simulink model "EHB_speedgoat_R2020a_V1"  (R2020a)
settings: Solver=FixedStepDiscrete  StartTime=0.0  StopTime=inf  FixedStep=0.001  RelTol=1e-3  EnableMultiTasking=on
model workspace (MAT data in the model file):
  A : Simulink.Signal (value not decoded)
  B : Simulink.Signal (value not decoded)
  C : Simulink.Signal (value not decoded)
  D : Simulink.Signal (value not decoded)
  E : Simulink.Signal (value not decoded)
  calin = [-9.96 -7.98 -5.98 -3.99 -1.994 0 1.995 3.992 5.99 7.98 9.97]
  calout = [-10 -8 -6 -4 -2 0 2 4 6 8 10]
symbols that are objects in the model workspace (value not decoded): C, D
undefined symbols (not defined in the file): Com1, none, ts_IO612
libraries: simulink x1436, xpcethercatlib x1223, yisutbxlib_utilities x256, xpcutilitieslib x156, hdlsllib x145, canmsglib x46, speedgoatlib_IO602_4 x11, speedgoatlib_IO611 x7, slrttcplib x4, CanManageLib x3, slrtlib x3, xpcseriallib x2
(part 6 of 30)

== system EHB_speedgoat_R2020a_V1/保留/YS4008/YS4008_M_1 ==
  note: 每路通道4种故障类型，同时最多只能有1个为1（软件保护），当一个通道同时注入超过一种故障时，会自动清除当前通道的所有故障，恢复默认模式。
  note: FIU_SetCH: 0 无故障
      | 1 短路到KL30
      | 2 短路到KL31
      | 4 共轨
      | 8 开路
  note: Rock表示插箱号，一般是0；
      |
      | Slot表示板卡的编号，由板卡上的拨码开关决定；
  FIU_SetCH{1..8} (8 alike) : Constant  Value=0  OutDataTypeStr=Inherit: Inherit via back propagation
  PassWord : Constant  Value=0xAA  OutDataTypeStr=uint8
  Rack : Constant  Value=0  OutDataTypeStr=uint8
  Slot : Constant  OutDataTypeStr=uint8
  YS4008_M : Subsystem
  tag scope: YS4008_M_1=global
  wires:
  PassWord/1 -> YS4008_M/1(PassWord)  "PassWord"
  Rack/1 -> YS4008_M/10(Rack)  "Rack"
  Slot/1 -> YS4008_M/11(Slot)  "Slot"
  FIU_SetCH4/1 -> YS4008_M/5(FIU_SetCH4)  "FIU_SetCH4"
  FIU_SetCH1/1 -> YS4008_M/2(FIU_SetCH1)  "FIU_SetCH1"
  FIU_SetCH8/1 -> YS4008_M/9(FIU_SetCH8)  "FIU_SetCH8"
  FIU_SetCH5/1 -> YS4008_M/6(FIU_SetCH5)  "FIU_SetCH5"
  FIU_SetCH3/1 -> YS4008_M/4(FIU_SetCH3)  "FIU_SetCH3"
  FIU_SetCH2/1 -> YS4008_M/3(FIU_SetCH2)  "FIU_SetCH2"
  FIU_SetCH6/1 -> YS4008_M/7(FIU_SetCH6)  "FIU_SetCH6"
  FIU_SetCH7/1 -> YS4008_M/8(FIU_SetCH7)  "FIU_SetCH7"
  YS4008_M/1(Output) -> [YS4008_M_1]

== system EHB_speedgoat_R2020a_V1/保留/YS4008/YS4008_M_2 ==
  note: Rock表示插箱号，一般是0；
      |
      | Slot表示板卡的编号，由板卡上的拨码开关决定；
  note: FIU_SetCH: 0 无故障
      | 1 短路到KL30
      | 2 短路到KL31
      | 4 共轨
      | 8 开路
  note: 每路通道4种故障类型，同时最多只能有1个为1（软件保护），当一个通道同时注入超过一种故障时，会自动清除当前通道的所有故障，恢复默认模式。
  FIU_SetCH{1..8} (8 alike) : Constant  Value=0  OutDataTypeStr=Inherit: Inherit via back propagation
  PassWord : Constant  Value=0xAA  OutDataTypeStr=uint8
  Rack : Constant  Value=0  OutDataTypeStr=uint8
  Slot : Constant  Value=2  OutDataTypeStr=uint8
  YS4008_M : Subsystem
  tag scope: YS4008_M_2=global
  wires:
  FIU_SetCH6/1 -> YS4008_M/7(FIU_SetCH6)  "FIU_SetCH6"
  FIU_SetCH3/1 -> YS4008_M/4(FIU_SetCH3)  "FIU_SetCH3"
  FIU_SetCH2/1 -> YS4008_M/3(FIU_SetCH2)  "FIU_SetCH2"
  FIU_SetCH1/1 -> YS4008_M/2(FIU_SetCH1)  "FIU_SetCH1"
  FIU_SetCH7/1 -> YS4008_M/8(FIU_SetCH7)  "FIU_SetCH7"
  FIU_SetCH4/1 -> YS4008_M/5(FIU_SetCH4)  "FIU_SetCH4"
  FIU_SetCH5/1 -> YS4008_M/6(FIU_SetCH5)  "FIU_SetCH5"
  FIU_SetCH8/1 -> YS4008_M/9(FIU_SetCH8)  "FIU_SetCH8"
  Slot/1 -> YS4008_M/11(Slot)  "Slot"
  PassWord/1 -> YS4008_M/1(PassWord)  "PassWord"
  Rack/1 -> YS4008_M/10(Rack)  "Rack"
  YS4008_M/1(Output) -> [YS4008_M_2]

== system EHB_speedgoat_R2020a_V1/保留/YS4008/YS4008_M_3 ==
  note: 每路通道4种故障类型，同时最多只能有1个为1（软件保护），当一个通道同时注入超过一种故障时，会自动清除当前通道的所有故障，恢复默认模式。
  note: FIU_SetCH: 0 无故障
      | 1 短路到KL30
      | 2 短路到KL31
      | 4 共轨
      | 8 开路
  note: Rock表示插箱号，一般是0；
      |
      | Slot表示板卡的编号，由板卡上的拨码开关决定；
  FIU_SetCH{1..8} (8 alike) : Constant  Value=0  OutDataTypeStr=Inherit: Inherit via back propagation
  PassWord : Constant  Value=0xAA  OutDataTypeStr=uint8
  Rack : Constant  Value=0  OutDataTypeStr=uint8
  Slot : Constant  Value=3  OutDataTypeStr=uint8
  YS4008_M : Subsystem
  tag scope: YS4008_M_3=global
  wires:
  Rack/1 -> YS4008_M/10(Rack)  "Rack"
  FIU_SetCH8/1 -> YS4008_M/9(FIU_SetCH8)  "FIU_SetCH8"
  Slot/1 -> YS4008_M/11(Slot)  "Slot"
  PassWord/1 -> YS4008_M/1(PassWord)  "PassWord"
  FIU_SetCH5/1 -> YS4008_M/6(FIU_SetCH5)  "FIU_SetCH5"
  FIU_SetCH3/1 -> YS4008_M/4(FIU_SetCH3)  "FIU_SetCH3"
  FIU_SetCH4/1 -> YS4008_M/5(FIU_SetCH4)  "FIU_SetCH4"
  FIU_SetCH2/1 -> YS4008_M/3(FIU_SetCH2)  "FIU_SetCH2"
  FIU_SetCH1/1 -> YS4008_M/2(FIU_SetCH1)  "FIU_SetCH1"
  FIU_SetCH7/1 -> YS4008_M/8(FIU_SetCH7)  "FIU_SetCH7"
  FIU_SetCH6/1 -> YS4008_M/7(FIU_SetCH6)  "FIU_SetCH6"
  YS4008_M/1(Output) -> [YS4008_M_3]

== system EHB_speedgoat_R2020a_V1/保留/YS4008/YS4008_M_4 ==
  note: Rock表示插箱号，一般是0；
      |
      | Slot表示板卡的编号，由板卡上的拨码开关决定；
  note: FIU_SetCH: 0 无故障
      | 1 短路到KL30
      | 2 短路到KL31
      | 4 共轨
      | 8 开路
  note: 每路通道4种故障类型，同时最多只能有1个为1（软件保护），当一个通道同时注入超过一种故障时，会自动清除当前通道的所有故障，恢复默认模式。
  FIU_SetCH{1..8} (8 alike) : Constant  Value=0  OutDataTypeStr=Inherit: Inherit via back propagation
  PassWord : Constant  Value=0xAA  OutDataTypeStr=uint8
  Rack : Constant  Value=0  OutDataTypeStr=uint8
  Slot : Constant  Value=4  OutDataTypeStr=uint8
  YS4008_M1 : Subsystem
  tag scope: YS4008_M_4=global
  wires:
  Rack/1 -> YS4008_M1/10(Rack)  "Rack"
  FIU_SetCH7/1 -> YS4008_M1/8(FIU_SetCH7)  "FIU_SetCH7"
  FIU_SetCH6/1 -> YS4008_M1/7(FIU_SetCH6)  "FIU_SetCH6"
  FIU_SetCH2/1 -> YS4008_M1/3(FIU_SetCH2)  "FIU_SetCH2"
  FIU_SetCH4/1 -> YS4008_M1/5(FIU_SetCH4)  "FIU_SetCH4"
  FIU_SetCH5/1 -> YS4008_M1/6(FIU_SetCH5)  "FIU_SetCH5"
  PassWord/1 -> YS4008_M1/1(PassWord)  "PassWord"
  FIU_SetCH3/1 -> YS4008_M1/4(FIU_SetCH3)  "FIU_SetCH3"
  Slot/1 -> YS4008_M1/11(Slot)  "Slot"
  FIU_SetCH1/1 -> YS4008_M1/2(FIU_SetCH1)  "FIU_SetCH1"
  FIU_SetCH8/1 -> YS4008_M1/9(FIU_SetCH8)  "FIU_SetCH8"
  YS4008_M1/1(Output) -> [YS4008_M_4]

== system EHB_speedgoat_R2020a_V1/保留/YS4008/YS4008_M_5 ==
  note: 每路通道4种故障类型，同时最多只能有1个为1（软件保护），当一个通道同时注入超过一种故障时，会自动清除当前通道的所有故障，恢复默认模式。
  note: FIU_SetCH: 0 无故障
      | 1 短路到KL30
      | 2 短路到KL31
      | 4 共轨
      | 8 开路
  note: Rock表示插箱号，一般是0；
      |
      | Slot表示板卡的编号，由板卡上的拨码开关决定；
  FIU_SetCH{1..8} (8 alike) : Constant  Value=0  OutDataTypeStr=Inherit: Inherit via back propagation
  PassWord : Constant  Value=0xAA  OutDataTypeStr=uint8
  Rack : Constant  Value=0  OutDataTypeStr=uint8
  Slot : Constant  Value=5  OutDataTypeStr=uint8
  YS4008_M : Subsystem
  tag scope: YS4008_M_5=global
  wires:
  FIU_SetCH1/1 -> YS4008_M/2(FIU_SetCH1)  "FIU_SetCH1"
  FIU_SetCH3/1 -> YS4008_M/4(FIU_SetCH3)  "FIU_SetCH3"
  FIU_SetCH5/1 -> YS4008_M/6(FIU_SetCH5)  "FIU_SetCH5"
  Slot/1 -> YS4008_M/11(Slot)  "Slot"
  PassWord/1 -> YS4008_M/1(PassWord)  "PassWord"
  FIU_SetCH4/1 -> YS4008_M/5(FIU_SetCH4)  "FIU_SetCH4"
  FIU_SetCH2/1 -> YS4008_M/3(FIU_SetCH2)  "FIU_SetCH2"
  FIU_SetCH6/1 -> YS4008_M/7(FIU_SetCH6)  "FIU_SetCH6"
  Rack/1 -> YS4008_M/10(Rack)  "Rack"
  FIU_SetCH7/1 -> YS4008_M/8(FIU_SetCH7)  "FIU_SetCH7"
  FIU_SetCH8/1 -> YS4008_M/9(FIU_SetCH8)  "FIU_SetCH8"
  YS4008_M/1(Output) -> [YS4008_M_5]

== system EHB_speedgoat_R2020a_V1/保留/YS4008/YS4008_M_6 ==
  note: Rock表示插箱号，一般是0；
      |
      | Slot表示板卡的编号，由板卡上的拨码开关决定；
  note: FIU_SetCH: 0 无故障
      | 1 短路到KL30
      | 2 短路到KL31
      | 4 共轨
      | 8 开路
  note: 每路通道4种故障类型，同时最多只能有1个为1（软件保护），当一个通道同时注入超过一种故障时，会自动清除当前通道的所有故障，恢复默认模式。
  FIU_SetCH{1..8} (8 alike) : Constant  Value=0  OutDataTypeStr=Inherit: Inherit via back propagation
  PassWord : Constant  Value=0xAA  OutDataTypeStr=uint8
  Rack : Constant  Value=0  OutDataTypeStr=uint8
  Slot : Constant  Value=6  OutDataTypeStr=uint8
  YS4008_M : Subsystem
  tag scope: YS4008_M_6=global
  wires:
  FIU_SetCH7/1 -> YS4008_M/8(FIU_SetCH7)  "FIU_SetCH7"
  Slot/1 -> YS4008_M/11(Slot)  "Slot"
  FIU_SetCH6/1 -> YS4008_M/7(FIU_SetCH6)  "FIU_SetCH6"
  FIU_SetCH2/1 -> YS4008_M/3(FIU_SetCH2)  "FIU_SetCH2"
  FIU_SetCH4/1 -> YS4008_M/5(FIU_SetCH4)  "FIU_SetCH4"
  Rack/1 -> YS4008_M/10(Rack)  "Rack"
  FIU_SetCH3/1 -> YS4008_M/4(FIU_SetCH3)  "FIU_SetCH3"
  FIU_SetCH5/1 -> YS4008_M/6(FIU_SetCH5)  "FIU_SetCH5"
  FIU_SetCH8/1 -> YS4008_M/9(FIU_SetCH8)  "FIU_SetCH8"
  FIU_SetCH1/1 -> YS4008_M/2(FIU_SetCH1)  "FIU_SetCH1"
  PassWord/1 -> YS4008_M/1(PassWord)  "PassWord"
  YS4008_M/1(Output) -> [YS4008_M_6]

== system EHB_speedgoat_R2020a_V1/保留/YS7501_M/HVRealy_Set ==
  RLY1 : Inport
  RLY2 : Inport  Port=2
  RLY3 : Inport  Port=3
  RLY4 : Inport  Port=4
  RLY5 : Inport  Port=5
  RLY6 : Inport  Port=6
  RLY7 : Inport  Port=7
  RLY8 : Inport  Port=8
  RLY9 : Inport  Port=9
  RLY10 : Inport  Port=10
  RLY11 : Inport  Port=11
  RLY12 : Inport  Port=12
  RLY13 : Inport  Port=13
  RLY14 : Inport  Port=14
  RLY15 : Inport  Port=15
  RLY16 : Inport  Port=16
  Trigger : TriggerPort  VariantControl=(inherit)  PortDimensions=1
  CAN Pack1 : canmsglib/CAN Pack  MsgList=(none)  MsgName=YS7501_M  MsgIDType=Standard (11-bit identifier)  MsgIdentifier=1856  MsgLength=8  Remote=off  ApplyMinMax=off  BusOutput=on  SignalInfo={ 'Rly1', '8', '1', 'BE', 'unsigned', 'Standard', '0', '1', '0', '0', '1'; 'Rly10', '17', '1', 'BE', 'unsigned', 'Standard', '0', '1', '0', '0', '1'; 'Rly11', '18', '1', 'BE', 'unsigned', 'Standard', '0', '1', '0', '0', '1'; 'Rly12', '19', '1', 'BE', 'unsigned', 'Standard', '0', '1', '0', '0', '1'; 'Rly13', '20', '1', 'BE', 'unsigned', 'Standard', '0', '1', '0', '0', '1'; 'Rly14', '21', '1', 'BE', 'unsigned', 'Standard', '0', '1', '0', '0', '1'; 'Rly15', '22', '1', 'BE', 'unsigned', 'Standard', '0', '1', '0', '0', '1'; 'Rly16', '23', '1', 'BE', 'unsigned', 'Standard', '0', '1', '0', '0', '1'; 'Rly2', '9', '1', 'BE', 'unsigned', 'Standard', '0', '1', '0', '0', '1'; 'Rly3', '10', '1', 'BE', 'unsigned', 'Standard', '0', '1', '0', '0', '1'; 'Rly4', '11', '1', 'BE', 'unsigned', 'Standard', '0', '1', '0', '0', '1'; 'Rly5', '12', '1', 'BE', 'unsigned', 'Standard', '0', '1', '0', '0', '1'; 'Rly6', '13', '1', 'BE', 'unsigned', 'Standard', '0', '1', '0', '0', '1'; 'Rly7', '14', '1', 'BE', 'unsigned', 'Standard', '0', '1', '0', '0', '1'; 'Rly8', '15', '1', 'BE', 'unsigned', 'Standard', '0', '1', '0', '0', '1'; 'Rly9', '16', '1', 'BE', 'unsigned', 'Standard', '0', '1', '0', '0', '1'; 'Rly_en', '0', '1', 'BE', 'unsigned', 'Standard', '0', '1', '0', '0', '1' }
      settings: SourceProductBaseCode=ME,VN  DataFormat=manually specified signals
  CANDataPack_ToUDP : Subsystem
  Constant : Constant
  Output : Outport
  wires:
  CAN Pack1/1 -> CANDataPack_ToUDP/1(In1)
  RLY1/1 -> CAN Pack1/1
  RLY2/1 -> CAN Pack1/9
  RLY3/1 -> CAN Pack1/10
  RLY4/1 -> CAN Pack1/11
  RLY5/1 -> CAN Pack1/12
  RLY6/1 -> CAN Pack1/13
  RLY7/1 -> CAN Pack1/14
  RLY8/1 -> CAN Pack1/15
  RLY9/1 -> CAN Pack1/16
  RLY14/1 -> CAN Pack1/6
  RLY13/1 -> CAN Pack1/5
  RLY12/1 -> CAN Pack1/4
  RLY11/1 -> CAN Pack1/3
  RLY10/1 -> CAN Pack1/2
  RLY15/1 -> CAN Pack1/7
  RLY16/1 -> CAN Pack1/8
  Constant/1 -> CAN Pack1/17
  CANDataPack_ToUDP/1(Output) -> Output/1

== system EHB_speedgoat_R2020a_V1/CAN_Send/CAN Transmit/VCU_Msg/VCU_BrakingRequest_0x120 ==
  VCU_BrakingRequest : Inport
  Enable : EnablePort
  Trigger : TriggerPort  VariantControl=Variant
  Bus Selector : BusSelector  OutputSignals=Brake_AimPressure,BrakingEnable,ParkingBrakeActive
  CAN Pack : canmsglib/CAN Pack  CANdbFile=F:\湖大艾盛\wushuadianji_20230612.dbc  MsgList=VCU_BrakingRequest  MsgName=VCU_BrakingRequest  MsgIDType=Standard (11-bit identifier)  MsgIdentifier=288  MsgLength=8  Remote=off  ApplyMinMax=off  BusOutput=on  SignalInfo={'Brake_AimPressure','8','8','BE','unsigned','Standard','0','0.1','0','-Inf','Inf';'BrakingEnable','0','4','BE','unsigned','Standard','0','1','0','-Inf','Inf';'ParkingBrakeActive','4','4','BE','unsigned','Standard','0','1','0','-Inf','Inf'}
      settings: SourceProductBaseCode=ME,VN  DataFormat=CANdb specified signals
  CAN Write : speedgoatlib_IO602_4/Legacy/CAN Write  id=1  ts=-1  channel=1  messageType=CAN  BusInput=on  enableStatusPort=off  canType=CAN (HS)  initValues=[602 1 -1 0 1 1 0 1]
      settings: SourceProductName=Simulink Real-Time: Speedgoat I/O Blockset
  sigSource1 : Subsystem
  sigSource2 : Subsystem
  sigSource3 : Subsystem
  wires:
  VCU_BrakingRequest/1 -> Bus Selector/1
  Bus Selector/1 -> sigSource1/1(InputSignal)  "<Brake_AimPressure>"
  sigSource1/1(OutputSignal) -> CAN Pack/1
  Bus Selector/2 -> sigSource2/1(InputSignal)  "<BrakingEnable>"
  sigSource2/1(OutputSignal) -> CAN Pack/2
  Bus Selector/3 -> sigSource3/1(InputSignal)  "<ParkingBrakeActive>"
  sigSource3/1(OutputSignal) -> CAN Pack/3
  CAN Pack/1 -> CAN Write/1

== system EHB_speedgoat_R2020a_V1/CAN_Send/Signal/CAN_Msg_VCU/VCU_BrakingRequest_0x120 ==
  Brake_AimPressure : Constant  Value=0
  BrakingEnable : Constant  Value=0
  Bus Creator : BusCreator  Inputs=3
  ParkingBrakeActive : Constant  Value=0
  dtc1 : DataTypeConversion
  dtc2 : DataTypeConversion
  dtc3 : DataTypeConversion
  VCU_BrakingRequest_0x120 : Outport
  wires:
  dtc1/1 -> Bus Creator/1  "Brake_AimPressure"
  Brake_AimPressure/1 -> dtc1/1  "Brake_AimPressure"
  dtc2/1 -> Bus Creator/2  "BrakingEnable"
  BrakingEnable/1 -> dtc2/1  "BrakingEnable"
  dtc3/1 -> Bus Creator/3  "ParkingBrakeActive"
  ParkingBrakeActive/1 -> dtc3/1  "ParkingBrakeActive"
  Bus Creator/1 -> VCU_BrakingRequest_0x120/1  "VCU_BrakingRequest_0x120"

== system EHB_speedgoat_R2020a_V1/CAN_Send/Trigger/Trigger_VCU_Msg/Trigger_VCU_BrakingRequest_0x120 ==
  note: 发送触发方式的拓展：
      | 1、循环周期发送(包括丢帧方式)；
      | 2、手动触发发送(增加调试模块)；
      | 3、待拓展模式；
  ConditionalTrigger : Ground
  Cycle : Subsystem
  Kick : Subsystem
  KickValueChange : Subsystem
      settings: OpenFcn=|
      | KickValuePath =[gcs,'/Kick/KickValue'];
      | KickValueTmp = str2num(get_param(KickValuePath,'Value'));
      | if KickValueTmp == 1
      | set_param(KickValuePath,'Value','0');
      | else
      | set_param(KickValuePath,'Value','1');
      | end
      | masKicks = Simulink.Mask.get(gcb);
      | DispKicks = sprintf('disp("KicksValue:%s")',get_param(KickValuePath,'Value'));
      | masKicks.Display = DispKicks;
      mask Display: disp("KicksValue:1")
  ModeSelect : Constant  Value=ModeSelect  SampleTime=-1
  Multiport Switch : MultiPortSwitch
  Out1 : Outport  VectorParamsAs1DForOutWhenUnconnected=off
  wires:
  ConditionalTrigger/1 -> Multiport Switch/4
  Multiport Switch/1 -> Out1/1
  ModeSelect/1 -> Multiport Switch/1
  Cycle/1(Out1) -> Multiport Switch/2
  Kick/1(Out1) -> Multiport Switch/3

== system EHB_speedgoat_R2020a_V1/PowerCtrl/PowerCtrl/CANOpenInit1/CANDataPack_ToUDP ==
  In1 : Inport
  "Bit Packing " : xpcutilitieslib/Bit Packing   MaskBitPatterns={[7],[6],[4 5],[0:3]}  MaskPackDataType=uint8  MaskPackDataSize=[1]
      settings: SourceProductBaseCode=XP
  Bit Slice : hdlsllib/Logic and Bit Operations/Bit Slice  lidx=3  ridx=0
      settings: SourceProductBaseCode=SL
  Bus Selector : BusSelector  OutputSignals=Extended,Length,Remote,ID,Data
  "Byte Packing " : xpcutilitieslib/Byte Packing   MaskPackedDataType=uint8  MaskUnpackedDataTypes={'uint32'}  MaskAlignment=1
  "Byte Reversal " : xpcutilitieslib/Byte Reversal   numInp=1
      settings: SourceProductBaseCode=XP
  Constant1 : Constant  Value=[0 0]
  Data Type Conversion1 : DataTypeConversion  OutDataTypeStr=boolean
  Data Type Conversion2 : DataTypeConversion  OutDataTypeStr=uint8
  Data Type Conversion9 : DataTypeConversion  OutDataTypeStr=boolean
  Mux : Mux  Inputs=3
  Output : Outport
  wires:
  Bus Selector/5 -> Mux/3  "<Data>"
  "Bit Packing "/1 -> Mux/1  "YS5002_PowerSet"
  Bus Selector/2 -> Data Type Conversion2/1  "<Length>"
  Bus Selector/4 -> "Byte Reversal "/1  "<ID>"
  In1/1 -> Bus Selector/1
  Bus Selector/1 -> Data Type Conversion9/1  "<Extended>"
  Bus Selector/3 -> Data Type Conversion1/1  "<Remote>"
  Data Type Conversion9/1 -> "Bit Packing "/1
  "Byte Reversal "/1 -> "Byte Packing "/1
  Bit Slice/1 -> "Bit Packing "/4
  "Byte Packing "/1 -> Mux/2
  Constant1/1 -> "Bit Packing "/3
  Mux/1 -> Output/1
  Data Type Conversion2/1 -> Bit Slice/1
  Data Type Conversion1/1 -> "Bit Packing "/2

== system EHB_speedgoat_R2020a_V1/PowerCtrl/PowerCtrl/CurrSet1/CANDataPack_ToUDP ==
  In1 : Inport
  "Bit Packing " : xpcutilitieslib/Bit Packing   MaskBitPatterns={[7],[6],[4 5],[0:3]}  MaskPackDataType=uint8  MaskPackDataSize=[1]
      settings: SourceProductBaseCode=XP
  Bit Slice : hdlsllib/Logic and Bit Operations/Bit Slice  lidx=3  ridx=0
      settings: SourceProductBaseCode=SL
  Bus Selector : BusSelector  OutputSignals=Extended,Length,Remote,ID,Data
  "Byte Packing " : xpcutilitieslib/Byte Packing   MaskPackedDataType=uint8  MaskUnpackedDataTypes={'uint32'}  MaskAlignment=1
  "Byte Reversal " : xpcutilitieslib/Byte Reversal   numInp=1
      settings: SourceProductBaseCode=XP
  Constant1 : Constant  Value=[0 0]
  Data Type Conversion1 : DataTypeConversion  OutDataTypeStr=boolean
  Data Type Conversion2 : DataTypeConversion  OutDataTypeStr=uint8
  Data Type Conversion9 : DataTypeConversion  OutDataTypeStr=boolean
  Mux : Mux  Inputs=3
  Output : Outport
  wires:
  Bus Selector/5 -> Mux/3  "<Data>"
  "Bit Packing "/1 -> Mux/1  "YS5002_PowerSet"
  Bus Selector/2 -> Data Type Conversion2/1  "<Length>"
  Bus Selector/4 -> "Byte Reversal "/1  "<ID>"
  In1/1 -> Bus Selector/1
  Bus Selector/1 -> Data Type Conversion9/1  "<Extended>"
  Bus Selector/3 -> Data Type Conversion1/1  "<Remote>"
  Data Type Conversion9/1 -> "Bit Packing "/1
  "Byte Reversal "/1 -> "Byte Packing "/1
  Bit Slice/1 -> "Bit Packing "/4
  "Byte Packing "/1 -> Mux/2
  Constant1/1 -> "Bit Packing "/3
  Mux/1 -> Output/1
  Data Type Conversion2/1 -> Bit Slice/1
  Data Type Conversion1/1 -> "Bit Packing "/2

== system EHB_speedgoat_R2020a_V1/PowerCtrl/PowerCtrl/Enable1/CANDataPack_ToUDP ==
  In1 : Inport
  "Bit Packing " : xpcutilitieslib/Bit Packing   MaskBitPatterns={[7],[6],[4 5],[0:3]}  MaskPackDataType=uint8  MaskPackDataSize=[1]
      settings: SourceProductBaseCode=XP
  Bit Slice : hdlsllib/Logic and Bit Operations/Bit Slice  lidx=3  ridx=0
      settings: SourceProductBaseCode=SL
  Bus Selector : BusSelector  OutputSignals=Extended,Length,Remote,ID,Data
  "Byte Packing " : xpcutilitieslib/Byte Packing   MaskPackedDataType=uint8  MaskUnpackedDataTypes={'uint32'}  MaskAlignment=1
  "Byte Reversal " : xpcutilitieslib/Byte Reversal   numInp=1
      settings: SourceProductBaseCode=XP
  Constant1 : Constant  Value=[0 0]
  Data Type Conversion1 : DataTypeConversion  OutDataTypeStr=boolean
  Data Type Conversion2 : DataTypeConversion  OutDataTypeStr=uint8
  Data Type Conversion9 : DataTypeConversion  OutDataTypeStr=boolean
  Mux : Mux  Inputs=3
  Output : Outport
  wires:
  Bus Selector/5 -> Mux/3  "<Data>"
  "Bit Packing "/1 -> Mux/1  "YS5002_PowerSet"
  Bus Selector/2 -> Data Type Conversion2/1  "<Length>"
  Bus Selector/4 -> "Byte Reversal "/1  "<ID>"
  In1/1 -> Bus Selector/1
  Bus Selector/1 -> Data Type Conversion9/1  "<Extended>"
  Bus Selector/3 -> Data Type Conversion1/1  "<Remote>"
  Data Type Conversion9/1 -> "Bit Packing "/1
  "Byte Reversal "/1 -> "Byte Packing "/1
  Bit Slice/1 -> "Bit Packing "/4
  "Byte Packing "/1 -> Mux/2
  Constant1/1 -> "Bit Packing "/3
  Mux/1 -> Output/1
  Data Type Conversion2/1 -> Bit Slice/1
  Data Type Conversion1/1 -> "Bit Packing "/2

== system EHB_speedgoat_R2020a_V1/PowerCtrl/PowerCtrl/PowerPosSet1/CANDataPack_ToUDP ==
  In1 : Inport
  "Bit Packing " : xpcutilitieslib/Bit Packing   MaskBitPatterns={[7],[6],[4 5],[0:3]}  MaskPackDataType=uint8  MaskPackDataSize=[1]
      settings: SourceProductBaseCode=XP
  Bit Slice : hdlsllib/Logic and Bit Operations/Bit Slice  lidx=3  ridx=0
      settings: SourceProductBaseCode=SL
  Bus Selector : BusSelector  OutputSignals=Extended,Length,Remote,ID,Data
  "Byte Packing " : xpcutilitieslib/Byte Packing   MaskPackedDataType=uint8  MaskUnpackedDataTypes={'uint32'}  MaskAlignment=1
  "Byte Reversal " : xpcutilitieslib/Byte Reversal   numInp=1
      settings: SourceProductBaseCode=XP
  Constant1 : Constant  Value=[0 0]
  Data Type Conversion1 : DataTypeConversion  OutDataTypeStr=boolean
  Data Type Conversion2 : DataTypeConversion  OutDataTypeStr=uint8
  Data Type Conversion9 : DataTypeConversion  OutDataTypeStr=boolean
  Mux : Mux  Inputs=3
  Output : Outport
  wires:
  Bus Selector/5 -> Mux/3  "<Data>"
  "Bit Packing "/1 -> Mux/1  "YS5002_PowerSet"
  Bus Selector/2 -> Data Type Conversion2/1  "<Length>"
  Bus Selector/4 -> "Byte Reversal "/1  "<ID>"
  In1/1 -> Bus Selector/1
  Bus Selector/1 -> Data Type Conversion9/1  "<Extended>"
  Bus Selector/3 -> Data Type Conversion1/1  "<Remote>"
  Data Type Conversion9/1 -> "Bit Packing "/1
  "Byte Reversal "/1 -> "Byte Packing "/1
  Bit Slice/1 -> "Bit Packing "/4
  "Byte Packing "/1 -> Mux/2
  Constant1/1 -> "Bit Packing "/3
  Mux/1 -> Output/1
  Data Type Conversion2/1 -> Bit Slice/1
  Data Type Conversion1/1 -> "Bit Packing "/2

== system EHB_speedgoat_R2020a_V1/PowerCtrl/PowerCtrl/VoltSet1/CANDataPack_ToUDP ==
  In1 : Inport
  "Bit Packing " : xpcutilitieslib/Bit Packing   MaskBitPatterns={[7],[6],[4 5],[0:3]}  MaskPackDataType=uint8  MaskPackDataSize=[1]
      settings: SourceProductBaseCode=XP
  Bit Slice : hdlsllib/Logic and Bit Operations/Bit Slice  lidx=3  ridx=0
      settings: SourceProductBaseCode=SL
  Bus Selector : BusSelector  OutputSignals=Extended,Length,Remote,ID,Data
  "Byte Packing " : xpcutilitieslib/Byte Packing   MaskPackedDataType=uint8  MaskUnpackedDataTypes={'uint32'}  MaskAlignment=1
  "Byte Reversal " : xpcutilitieslib/Byte Reversal   numInp=1
      settings: SourceProductBaseCode=XP
  Constant1 : Constant  Value=[0 0]
  Data Type Conversion1 : DataTypeConversion  OutDataTypeStr=boolean
  Data Type Conversion2 : DataTypeConversion  OutDataTypeStr=uint8
  Data Type Conversion9 : DataTypeConversion  OutDataTypeStr=boolean
  Mux : Mux  Inputs=3
  Output : Outport
  wires:
  Bus Selector/5 -> Mux/3  "<Data>"
  "Bit Packing "/1 -> Mux/1  "YS5002_PowerSet"
  Bus Selector/2 -> Data Type Conversion2/1  "<Length>"
  Bus Selector/4 -> "Byte Reversal "/1  "<ID>"
  In1/1 -> Bus Selector/1
  Bus Selector/1 -> Data Type Conversion9/1  "<Extended>"
  Bus Selector/3 -> Data Type Conversion1/1  "<Remote>"
  Data Type Conversion9/1 -> "Bit Packing "/1
  "Byte Reversal "/1 -> "Byte Packing "/1
  Bit Slice/1 -> "Bit Packing "/4
  "Byte Packing "/1 -> Mux/2
  Constant1/1 -> "Bit Packing "/3
  Mux/1 -> Output/1
  Data Type Conversion2/1 -> Bit Slice/1
  Data Type Conversion1/1 -> "Bit Packing "/2

== system EHB_speedgoat_R2020a_V1/TIF_04/CB2020_1/DAC1/dp2c CH1 ==
  dac_value : Inport
  dac_value_calibrate : Inport  Port=2
  Add : Sum
  Add1 : Sum
  Constant : Constant  Value=0
  Data Type Conversion : DataTypeConversion  OutDataTypeStr=int16
  Gain : Gain  Gain=32767/15
  Gain1 : Gain
  Saturation : Saturate  UpperLimit=12  LowerLimit=-12
  cmd_value : Outport
  wires:
  Gain/1 -> Add1/1
  Saturation/1 -> Add/1
  dac_value_calibrate/1 -> Add1/2
  dac_value/1 -> Gain1/1
  Constant/1 -> Add/2
  Add/1 -> Gain/1
  Data Type Conversion/1 -> cmd_value/1
  Add1/1 -> Data Type Conversion/1
  Gain1/1 -> Saturation/1

== system EHB_speedgoat_R2020a_V1/TIF_04/CB2020_2/DAC/dp2c CH1 ==
  dac_value : Inport
  dac_value_calibrate : Inport  Port=2
  Add : Sum
  Add1 : Sum
  Constant : Constant  Value=0
  Data Type Conversion : DataTypeConversion
  Gain : Gain  Gain=32767/15
  Gain1 : Gain
  Saturation : Saturate  UpperLimit=12  LowerLimit=-12
  cmd_value : Outport
  wires:
  Gain/1 -> Add1/1
  Saturation/1 -> Add/1
  dac_value_calibrate/1 -> Add1/2
  dac_value/1 -> Gain1/1
  Constant/1 -> Add/2
  Add/1 -> Gain/1
  Data Type Conversion/1 -> cmd_value/1
  Add1/1 -> Data Type Conversion/1
  Gain1/1 -> Saturation/1

== system EHB_speedgoat_R2020a_V1/TIF_04/CB2020_2/DAC/dp2c CH10 ==
  dac_value : Inport
  dac_value_calibrate : Inport  Port=2
  Add : Sum
  Add1 : Sum
  Constant : Constant  Value=0
  Data Type Conversion : DataTypeConversion
  Gain : Gain  Gain=32767/15
  Gain1 : Gain
  Saturation : Saturate  UpperLimit=12  LowerLimit=-12
  cmd_value : Outport
  wires:
  Gain/1 -> Add1/1
  Saturation/1 -> Add/1
  dac_value_calibrate/1 -> Add1/2
  dac_value/1 -> Gain1/1
  Constant/1 -> Add/2
  Add/1 -> Gain/1
  Data Type Conversion/1 -> cmd_value/1
  Add1/1 -> Data Type Conversion/1
  Gain1/1 -> Saturation/1

== system EHB_speedgoat_R2020a_V1/TIF_04/CB2020_2/DAC/dp2c CH11 ==
  dac_value : Inport
  dac_value_calibrate : Inport  Port=2
  Add : Sum
  Add1 : Sum
  Constant : Constant  Value=0
  Data Type Conversion : DataTypeConversion
  Gain : Gain  Gain=32767/15
  Gain1 : Gain
  Saturation : Saturate  UpperLimit=12  LowerLimit=-12
  cmd_value : Outport
  wires:
  Gain/1 -> Add1/1
  Saturation/1 -> Add/1
  dac_value_calibrate/1 -> Add1/2
  dac_value/1 -> Gain1/1
  Constant/1 -> Add/2
  Add/1 -> Gain/1
  Data Type Conversion/1 -> cmd_value/1
  Add1/1 -> Data Type Conversion/1
  Gain1/1 -> Saturation/1

== system EHB_speedgoat_R2020a_V1/TIF_04/CB2020_2/DAC/dp2c CH12 ==
  dac_value : Inport
  dac_value_calibrate : Inport  Port=2
  Add : Sum
  Add1 : Sum
  Constant : Constant  Value=0
  Data Type Conversion : DataTypeConversion
  Gain : Gain  Gain=32767/15
  Gain1 : Gain
  Saturation : Saturate  UpperLimit=12  LowerLimit=-12
  cmd_value : Outport
  wires:
  Gain/1 -> Add1/1
  Saturation/1 -> Add/1
  dac_value_calibrate/1 -> Add1/2
  dac_value/1 -> Gain1/1
  Constant/1 -> Add/2
  Add/1 -> Gain/1
  Data Type Conversion/1 -> cmd_value/1
  Add1/1 -> Data Type Conversion/1
  Gain1/1 -> Saturation/1

== system EHB_speedgoat_R2020a_V1/TIF_04/CB2020_2/DAC/dp2c CH13 ==
  dac_value : Inport
  dac_value_calibrate : Inport  Port=2
  Add : Sum
  Add1 : Sum
  Constant : Constant  Value=0
  Data Type Conversion : DataTypeConversion
  Gain : Gain  Gain=32767/15
  Gain1 : Gain
  Saturation : Saturate  UpperLimit=12  LowerLimit=-12
  cmd_value : Outport
  wires:
  Gain/1 -> Add1/1
  Saturation/1 -> Add/1
  dac_value_calibrate/1 -> Add1/2
  dac_value/1 -> Gain1/1
  Constant/1 -> Add/2
  Add/1 -> Gain/1
  Data Type Conversion/1 -> cmd_value/1
  Add1/1 -> Data Type Conversion/1
  Gain1/1 -> Saturation/1

== system EHB_speedgoat_R2020a_V1/TIF_04/CB2020_2/DAC/dp2c CH14 ==
  dac_value : Inport
  dac_value_calibrate : Inport  Port=2
  Add : Sum
  Add1 : Sum
  Constant : Constant  Value=0
  Data Type Conversion : DataTypeConversion
  Gain : Gain  Gain=32767/15
  Gain1 : Gain
  Saturation : Saturate  UpperLimit=12  LowerLimit=-12
  cmd_value : Outport
  wires:
  Gain/1 -> Add1/1
  Saturation/1 -> Add/1
  dac_value_calibrate/1 -> Add1/2
  dac_value/1 -> Gain1/1
  Constant/1 -> Add/2
  Add/1 -> Gain/1
  Data Type Conversion/1 -> cmd_value/1
  Add1/1 -> Data Type Conversion/1
  Gain1/1 -> Saturation/1

== system EHB_speedgoat_R2020a_V1/TIF_04/CB2020_2/DAC/dp2c CH15 ==
  dac_value : Inport
  dac_value_calibrate : Inport  Port=2
  Add : Sum
  Add1 : Sum
  Constant : Constant  Value=0
  Data Type Conversion : DataTypeConversion
  Gain : Gain  Gain=32767/15
  Gain1 : Gain
  Saturation : Saturate  UpperLimit=12  LowerLimit=-12
  cmd_value : Outport
  wires:
  Gain/1 -> Add1/1
  Saturation/1 -> Add/1
  dac_value_calibrate/1 -> Add1/2
  dac_value/1 -> Gain1/1
  Constant/1 -> Add/2
  Add/1 -> Gain/1
  Data Type Conversion/1 -> cmd_value/1
  Add1/1 -> Data Type Conversion/1
  Gain1/1 -> Saturation/1

== system EHB_speedgoat_R2020a_V1/TIF_04/CB2020_2/DAC/dp2c CH16 ==
  dac_value : Inport
  dac_value_calibrate : Inport  Port=2
  Add : Sum
  Add1 : Sum
  Constant : Constant  Value=0
  Data Type Conversion : DataTypeConversion
  Gain : Gain  Gain=32767/15
  Gain1 : Gain
  Saturation : Saturate  UpperLimit=12  LowerLimit=-12
  cmd_value : Outport
  wires:
  Gain/1 -> Add1/1
  Saturation/1 -> Add/1
  dac_value_calibrate/1 -> Add1/2
  dac_value/1 -> Gain1/1
  Constant/1 -> Add/2
  Add/1 -> Gain/1
  Data Type Conversion/1 -> cmd_value/1
  Add1/1 -> Data Type Conversion/1
  Gain1/1 -> Saturation/1

== system EHB_speedgoat_R2020a_V1/TIF_04/CB2020_2/DAC/dp2c CH17 ==
  dac_value : Inport
  dac_value_calibrate : Inport  Port=2
  Add : Sum
  Add1 : Sum
  Constant : Constant  Value=0
  Data Type Conversion : DataTypeConversion
  Gain : Gain  Gain=32767/10
  Gain1 : Gain
  Saturation : Saturate  UpperLimit=10  LowerLimit=-10
  cmd_value : Outport
  wires:
  Gain/1 -> Add1/1
  Saturation/1 -> Add/1
  dac_value_calibrate/1 -> Add1/2
  dac_value/1 -> Gain1/1
  Constant/1 -> Add/2
  Add/1 -> Gain/1
  Data Type Conversion/1 -> cmd_value/1
  Add1/1 -> Data Type Conversion/1
  Gain1/1 -> Saturation/1

== system EHB_speedgoat_R2020a_V1/TIF_04/CB2020_2/DAC/dp2c CH18 ==
  dac_value : Inport
  dac_value_calibrate : Inport  Port=2
  Add : Sum
  Add1 : Sum
  Constant : Constant  Value=0
  Data Type Conversion : DataTypeConversion
  Gain : Gain  Gain=32767/10
  Gain1 : Gain
  Saturation : Saturate  UpperLimit=10  LowerLimit=-10
  cmd_value : Outport
  wires:
  Gain/1 -> Add1/1
  Saturation/1 -> Add/1
  dac_value_calibrate/1 -> Add1/2
  dac_value/1 -> Gain1/1
  Constant/1 -> Add/2
  Add/1 -> Gain/1
  Data Type Conversion/1 -> cmd_value/1
  Add1/1 -> Data Type Conversion/1
  Gain1/1 -> Saturation/1

== system EHB_speedgoat_R2020a_V1/TIF_04/CB2020_2/DAC/dp2c CH19 ==
  dac_value : Inport
  dac_value_calibrate : Inport  Port=2
  Add : Sum
  Add1 : Sum
  Constant : Constant  Value=0
  Data Type Conversion : DataTypeConversion
  Gain : Gain  Gain=32767/10
  Gain1 : Gain
  Saturation : Saturate  UpperLimit=10  LowerLimit=-10
  cmd_value : Outport
  wires:
  Gain/1 -> Add1/1
  Saturation/1 -> Add/1
  dac_value_calibrate/1 -> Add1/2
  dac_value/1 -> Gain1/1
  Constant/1 -> Add/2
  Add/1 -> Gain/1
  Data Type Conversion/1 -> cmd_value/1
  Add1/1 -> Data Type Conversion/1
  Gain1/1 -> Saturation/1

== system EHB_speedgoat_R2020a_V1/TIF_04/CB2020_2/DAC/dp2c CH2 ==
  dac_value : Inport
  dac_value_calibrate : Inport  Port=2
  Add : Sum
  Add1 : Sum
  Constant : Constant  Value=0
  Data Type Conversion : DataTypeConversion
  Gain : Gain  Gain=32767/15
  Gain1 : Gain
  Saturation : Saturate  UpperLimit=12  LowerLimit=-12
  cmd_value : Outport
  wires:
  Gain/1 -> Add1/1
  Saturation/1 -> Add/1
  dac_value_calibrate/1 -> Add1/2
  dac_value/1 -> Gain1/1
  Constant/1 -> Add/2
  Add/1 -> Gain/1
  Data Type Conversion/1 -> cmd_value/1
  Add1/1 -> Data Type Conversion/1
  Gain1/1 -> Saturation/1

== system EHB_speedgoat_R2020a_V1/TIF_04/CB2020_2/DAC/dp2c CH20 ==
  dac_value : Inport
  dac_value_calibrate : Inport  Port=2
  Add : Sum
  Add1 : Sum
  Constant : Constant  Value=0
  Data Type Conversion : DataTypeConversion
  Gain : Gain  Gain=32767/10
  Gain1 : Gain
  Saturation : Saturate  UpperLimit=10  LowerLimit=-10
  cmd_value : Outport
  wires:
  Gain/1 -> Add1/1
  Saturation/1 -> Add/1
  dac_value_calibrate/1 -> Add1/2
  dac_value/1 -> Gain1/1
  Constant/1 -> Add/2
  Add/1 -> Gain/1
  Data Type Conversion/1 -> cmd_value/1
  Add1/1 -> Data Type Conversion/1
  Gain1/1 -> Saturation/1

== system EHB_speedgoat_R2020a_V1/TIF_04/CB2020_2/DAC/dp2c CH3 ==
  dac_value : Inport
  dac_value_calibrate : Inport  Port=2
  Add : Sum
  Add1 : Sum
  Constant : Constant  Value=0
  Data Type Conversion : DataTypeConversion
  Gain : Gain  Gain=32767/15
  Gain1 : Gain
  Saturation : Saturate  UpperLimit=12  LowerLimit=-12
  cmd_value : Outport
  wires:
  Gain/1 -> Add1/1
  Saturation/1 -> Add/1
  dac_value_calibrate/1 -> Add1/2
  dac_value/1 -> Gain1/1
  Constant/1 -> Add/2
  Add/1 -> Gain/1
  Data Type Conversion/1 -> cmd_value/1
  Add1/1 -> Data Type Conversion/1
  Gain1/1 -> Saturation/1

== system EHB_speedgoat_R2020a_V1/TIF_04/CB2020_2/DAC/dp2c CH4 ==
  dac_value : Inport
  dac_value_calibrate : Inport  Port=2
  Add : Sum
  Add1 : Sum
  Constant : Constant  Value=0
  Data Type Conversion : DataTypeConversion
  Gain : Gain  Gain=32767/15
  Gain1 : Gain
  Saturation : Saturate  UpperLimit=12  LowerLimit=-12
  cmd_value : Outport
  wires:
  Gain/1 -> Add1/1
  Saturation/1 -> Add/1
  dac_value_calibrate/1 -> Add1/2
  dac_value/1 -> Gain1/1
  Constant/1 -> Add/2
  Add/1 -> Gain/1
  Data Type Conversion/1 -> cmd_value/1
  Add1/1 -> Data Type Conversion/1
  Gain1/1 -> Saturation/1

== system EHB_speedgoat_R2020a_V1/TIF_04/CB2020_2/DAC/dp2c CH5 ==
  dac_value : Inport
  dac_value_calibrate : Inport  Port=2
  Add : Sum
  Add1 : Sum
  Constant : Constant  Value=0
  Data Type Conversion : DataTypeConversion
  Gain : Gain  Gain=32767/15
  Gain1 : Gain
  Saturation : Saturate  UpperLimit=12  LowerLimit=-12
  cmd_value : Outport
  wires:
  Gain/1 -> Add1/1
  Saturation/1 -> Add/1
  dac_value_calibrate/1 -> Add1/2
  dac_value/1 -> Gain1/1
  Constant/1 -> Add/2
  Add/1 -> Gain/1
  Data Type Conversion/1 -> cmd_value/1
  Add1/1 -> Data Type Conversion/1
  Gain1/1 -> Saturation/1

== system EHB_speedgoat_R2020a_V1/TIF_04/CB2020_2/DAC/dp2c CH6 ==
  dac_value : Inport
  dac_value_calibrate : Inport  Port=2
  Add : Sum
  Add1 : Sum
  Constant : Constant  Value=0
  Data Type Conversion : DataTypeConversion
  Gain : Gain  Gain=32767/15
  Gain1 : Gain
  Saturation : Saturate  UpperLimit=12  LowerLimit=-12
  cmd_value : Outport
  wires:
  Gain/1 -> Add1/1
  Saturation/1 -> Add/1
  dac_value_calibrate/1 -> Add1/2
  dac_value/1 -> Gain1/1
  Constant/1 -> Add/2
  Add/1 -> Gain/1
  Data Type Conversion/1 -> cmd_value/1
  Add1/1 -> Data Type Conversion/1
  Gain1/1 -> Saturation/1

== system EHB_speedgoat_R2020a_V1/TIF_04/CB2020_2/DAC/dp2c CH7 ==
  dac_value : Inport
  dac_value_calibrate : Inport  Port=2
  Add : Sum
  Add1 : Sum
  Constant : Constant  Value=0
  Data Type Conversion : DataTypeConversion
  Gain : Gain  Gain=32767/15
  Gain1 : Gain
  Saturation : Saturate  UpperLimit=12  LowerLimit=-12
  cmd_value : Outport
  wires:
  Gain/1 -> Add1/1
  Saturation/1 -> Add/1
  dac_value_calibrate/1 -> Add1/2
  dac_value/1 -> Gain1/1
  Constant/1 -> Add/2
  Add/1 -> Gain/1
  Data Type Conversion/1 -> cmd_value/1
  Add1/1 -> Data Type Conversion/1
  Gain1/1 -> Saturation/1

== system EHB_speedgoat_R2020a_V1/TIF_04/CB2020_2/DAC/dp2c CH8 ==
  dac_value : Inport
  dac_value_calibrate : Inport  Port=2
  Add : Sum
  Add1 : Sum
  Constant : Constant  Value=0
  Data Type Conversion : DataTypeConversion
  Gain : Gain  Gain=32767/15
  Gain1 : Gain
  Saturation : Saturate  UpperLimit=12  LowerLimit=-12
  cmd_value : Outport
  wires:
  Gain/1 -> Add1/1
  Saturation/1 -> Add/1
  dac_value_calibrate/1 -> Add1/2
  dac_value/1 -> Gain1/1
  Constant/1 -> Add/2
  Add/1 -> Gain/1
  Data Type Conversion/1 -> cmd_value/1
  Add1/1 -> Data Type Conversion/1
  Gain1/1 -> Saturation/1

== system EHB_speedgoat_R2020a_V1/TIF_04/CB2020_2/DAC/dp2c CH9 ==
  dac_value : Inport
  dac_value_calibrate : Inport  Port=2
  Add : Sum
  Add1 : Sum
  Constant : Constant  Value=0
  Data Type Conversion : DataTypeConversion
  Gain : Gain  Gain=32767/15
  Gain1 : Gain
  Saturation : Saturate  UpperLimit=12  LowerLimit=-12
  cmd_value : Outport
  wires:
  Gain/1 -> Add1/1
  Saturation/1 -> Add/1
  dac_value_calibrate/1 -> Add1/2
  dac_value/1 -> Gain1/1
  Constant/1 -> Add/2
  Add/1 -> Gain/1
  Data Type Conversion/1 -> cmd_value/1
  Add1/1 -> Data Type Conversion/1
  Gain1/1 -> Saturation/1

== system EHB_speedgoat_R2020a_V1/TIF_04/CB2020_3/DAC1/dp2c CH1 ==
  dac_value : Inport
  dac_value_calibrate : Inport  Port=2
  Add : Sum
  Add1 : Sum
  Constant : Constant  Value=0
  Data Type Conversion : DataTypeConversion  OutDataTypeStr=int16
  Gain : Gain  Gain=32767/15
  Gain1 : Gain
  Saturation : Saturate  UpperLimit=12  LowerLimit=-12
  cmd_value : Outport
  wires:
  Gain/1 -> Add1/1
  Saturation/1 -> Add/1
  dac_value_calibrate/1 -> Add1/2
  dac_value/1 -> Gain1/1
  Constant/1 -> Add/2
  Add/1 -> Gain/1
  Data Type Conversion/1 -> cmd_value/1
  Add1/1 -> Data Type Conversion/1
  Gain1/1 -> Saturation/1

== system EHB_speedgoat_R2020a_V1/保留/TIF_01/YS4020_M_2/YS4020_M ==
  FIU_SetCH1 : Inport
  FIU_SetCH2 : Inport  Port=2
  FIU_SetCH3 : Inport  Port=3
  FIU_SetCH4 : Inport  Port=4
  FIU_SetCH5 : Inport  Port=5
  FIU_SetCH6 : Inport  Port=6
  FIU_SetCH7 : Inport  Port=7
  FIU_SetCH8 : Inport  Port=8
  FIU_SetCH9 : Inport  Port=9
  FIU_SetCH10 : Inport  Port=10
  FIU_SetCH11 : Inport  Port=11
  FIU_SetCH12 : Inport  Port=12
  FIU_SetCH13 : Inport  Port=13
  FIU_SetCH14 : Inport  Port=14
  FIU_SetCH15 : Inport  Port=15
  FIU_SetCH16 : Inport  Port=16
  FIU_SetCH17 : Inport  Port=17
  FIU_SetCH18 : Inport  Port=18
  FIU_SetCH19 : Inport  Port=19
  FIU_SetCH20 : Inport  Port=20
  PassWord : Inport  Port=21
  YS4020_M_Slot : Inport  Port=22
  Bus Creator : BusCreator  Inputs=12
  Bus Creator1 : BusCreator  Inputs=12
  Demux : Demux  Outputs=10
  Demux1 : Demux  Outputs=10
  FIU_CH1 : Subsystem
  FIU_CH10 : Subsystem
  FIU_CH11 : Subsystem
  FIU_CH12 : Subsystem
  FIU_CH13 : Subsystem
  FIU_CH14 : Subsystem
  FIU_CH15 : Subsystem
  FIU_CH16 : Subsystem
  FIU_CH17 : Subsystem
  FIU_CH18 : Subsystem
  FIU_CH19 : Subsystem
  FIU_CH2 : Subsystem
  FIU_CH20 : Subsystem
  FIU_CH3 : Subsystem
  FIU_CH4 : Subsystem
  FIU_CH5 : Subsystem
  FIU_CH6 : Subsystem
  FIU_CH7 : Subsystem
  FIU_CH8 : Subsystem
  FIU_CH9 : Subsystem
  FIU_MsgSend : Subsystem
  FIU_MsgSend1 : Subsystem
  Mux : Mux  Inputs=10
  Mux1 : Mux  Inputs=10
  YS4020_M_Ctrl_Trigger : Subsystem
  YS4020_M_Ctrl_Trigger1 : Subsystem
  tag scope: YS4020_M_2_1=global, YS4020_M_2_2=global
  wires:
  Mux1/1 -> [CH11_20], Demux1/1
  Demux1/1 -> FIU_CH11/1(FIU_SetCH1)
  YS4020_M_Ctrl_Trigger1/1(YS4020_M_CtrlTrigger) -> FIU_MsgSend1/Enable  "Trigger"
  Demux1/2 -> FIU_CH13/1(FIU_SetCH2)
  Demux1/3 -> FIU_CH14/1(FIU_SetCH3)
  Demux1/4 -> FIU_CH15/1(FIU_SetCH4)
  Demux1/5 -> FIU_CH16/1(FIU_SetCH5)
  Demux1/6 -> FIU_CH17/1(FIU_SetCH6)
  Demux1/7 -> FIU_CH18/1(FIU_SetCH7)
  Demux1/8 -> FIU_CH19/1(FIU_SetCH8)
  Demux1/9 -> FIU_CH20/1(FIU_SetCH9)
  Demux1/10 -> FIU_CH12/1(FIU_SetCH10)
  FIU_CH11/1(CH1_Out) -> Bus Creator1/3  "CH1_Out"
  FIU_CH13/1(CH2_Out) -> Bus Creator1/4  "CH2_Out"
  FIU_CH14/1(CH3_Out) -> Bus Creator1/5  "CH3_Out"
  FIU_CH15/1(CH4_Out) -> Bus Creator1/6  "CH4_Out"
  FIU_CH16/1(CH5_Out) -> Bus Creator1/7  "CH5_Out"
  FIU_CH17/1(CH6_Out) -> Bus Creator1/8  "CH6_Out"
  FIU_CH18/1(CH7_Out) -> Bus Creator1/9  "CH7_Out"
  FIU_CH19/1(CH8_Out) -> Bus Creator1/10  "CH8_Out"
  FIU_CH20/1(CH9_Out) -> Bus Creator1/11  "CH9_Out"
  FIU_CH12/1(CH10_Out) -> Bus Creator1/12  "CH10_Out"
  [CH11_20] -> YS4020_M_Ctrl_Trigger1/1(CH11_20)
  Bus Creator1/1 -> FIU_MsgSend1/1(YS4020_M)  "YS4020_M"
  [PassWord] -> Bus Creator1/1
  [Slot] -> Bus Creator1/2
  [Slot] -> Bus Creator/2
  [PassWord] -> Bus Creator/1
  PassWord/1 -> [PassWord]  "PassWord"
  YS4020_M_Slot/1 -> [Slot]  "YS4020_M_Slot"
  Bus Creator/1 -> FIU_MsgSend/1(YS4020_M)  "YS4020_M"
  [CH1_10] -> YS4020_M_Ctrl_Trigger/1(CH1_10)
  FIU_CH10/1(CH10_Out) -> Bus Creator/12  "CH10_Out"
  FIU_CH9/1(CH9_Out) -> Bus Creator/11  "CH9_Out"
  FIU_CH8/1(CH8_Out) -> Bus Creator/10  "CH8_Out"
  FIU_CH7/1(CH7_Out) -> Bus Creator/9  "CH7_Out"
  FIU_CH6/1(CH6_Out) -> Bus Creator/8  "CH6_Out"
  FIU_CH5/1(CH5_Out) -> Bus Creator/7  "CH5_Out"
  FIU_CH4/1(CH4_Out) -> Bus Creator/6  "CH4_Out"
  FIU_CH3/1(CH3_Out) -> Bus Creator/5  "CH3_Out"
  FIU_CH2/1(CH2_Out) -> Bus Creator/4  "CH2_Out"
  FIU_CH1/1(CH1_Out) -> Bus Creator/3  "CH1_Out"
  Demux/10 -> FIU_CH10/1(FIU_SetCH10)
  Demux/9 -> FIU_CH9/1(FIU_SetCH9)
  Demux/8 -> FIU_CH8/1(FIU_SetCH8)
  Demux/7 -> FIU_CH7/1(FIU_SetCH7)
  Demux/6 -> FIU_CH6/1(FIU_SetCH6)
  Demux/5 -> FIU_CH5/1(FIU_SetCH5)
  Demux/4 -> FIU_CH4/1(FIU_SetCH4)
  Demux/3 -> FIU_CH3/1(FIU_SetCH3)
  Demux/2 -> FIU_CH2/1(FIU_SetCH2)
  YS4020_M_Ctrl_Trigger/1(YS4020_M_CtrlTrigger) -> FIU_MsgSend/Enable  "Trigger"
  Demux/1 -> FIU_CH1/1(FIU_SetCH1)
  Mux/1 -> [CH1_10], Demux/1
  FIU_SetCH20/1 -> Mux1/10
  FIU_SetCH19/1 -> Mux1/9
  FIU_SetCH18/1 -> Mux1/8
  FIU_SetCH17/1 -> Mux1/7
  FIU_SetCH16/1 -> Mux1/6
  FIU_SetCH15/1 -> Mux1/5
  FIU_SetCH14/1 -> Mux1/4
  FIU_SetCH13/1 -> Mux1/3
  FIU_SetCH12/1 -> Mux1/2
  FIU_SetCH11/1 -> Mux1/1
  FIU_SetCH10/1 -> Mux/10
  FIU_SetCH9/1 -> Mux/9
  FIU_SetCH8/1 -> Mux/8
  FIU_SetCH7/1 -> Mux/7
  FIU_SetCH6/1 -> Mux/6
  FIU_SetCH5/1 -> Mux/5
  FIU_SetCH4/1 -> Mux/4
  FIU_SetCH3/1 -> Mux/3
  FIU_SetCH2/1 -> Mux/2
  FIU_SetCH1/1 -> Mux/1
  FIU_MsgSend/1(Output) -> [YS4020_M_2_1]
  FIU_MsgSend1/1(Output) -> [YS4020_M_2_2]

== system EHB_speedgoat_R2020a_V1/保留/TIF_02/CB3012_01/G2 RES ==
  Res_CH1 : Inport
  Res_CH2 : Inport  Port=2
  Res_CH3 : Inport  Port=3
  Res_CH4 : Inport  Port=4
  Res_CH5 : Inport  Port=5
  Res_CH6 : Inport  Port=6
  Res_CH7 : Inport  Port=7
  Res_CH8 : Inport  Port=8
  Res_CH9 : Inport  Port=9
  Res_CH10 : Inport  Port=10
  Res_CH11 : Inport  Port=11
  Res_CH12 : Inport  Port=12
  DTCB CH{1..12} (12 alike) : DataTypeConversion
  EtherCAT PDO Transmit RES CH1 : xpcethercatlib/EtherCAT PDO Transmit   Priority=3  sig_name=Box 8 (YISUWORLD).Setpoint Values process data mapping.ResValue1  sig_offset=12496  sig_type=uint16  type_size=16  sig_dim=1  device_id=0  sample_time=0.001000
      settings: SourceProductBaseCode=XP
  EtherCAT PDO Transmit RES CH10 : xpcethercatlib/EtherCAT PDO Transmit   Priority=3  sig_name=Box 8 (YISUWORLD).Setpoint Values process data mapping.ResValue10  sig_offset=12640  sig_type=uint16  type_size=16  sig_dim=1  device_id=0  sample_time=0.001000
      settings: SourceProductBaseCode=XP
  EtherCAT PDO Transmit RES CH11 : xpcethercatlib/EtherCAT PDO Transmit   Priority=3  sig_name=Box 8 (YISUWORLD).Setpoint Values process data mapping.ResValue11  sig_offset=12656  sig_type=uint16  type_size=16  sig_dim=1  device_id=0  sample_time=0.001000
      settings: SourceProductBaseCode=XP
  EtherCAT PDO Transmit RES CH12 : xpcethercatlib/EtherCAT PDO Transmit   Priority=3  sig_name=Box 8 (YISUWORLD).Setpoint Values process data mapping.ResValue12  sig_offset=12672  sig_type=uint16  type_size=16  sig_dim=1  device_id=0  sample_time=0.001000
      settings: SourceProductBaseCode=XP
  EtherCAT PDO Transmit RES CH2 : xpcethercatlib/EtherCAT PDO Transmit   Priority=3  sig_name=Box 8 (YISUWORLD).Setpoint Values process data mapping.ResValue2  sig_offset=12512  sig_type=uint16  type_size=16  sig_dim=1  device_id=0  sample_time=0.001000
      settings: SourceProductBaseCode=XP
  EtherCAT PDO Transmit RES CH3 : xpcethercatlib/EtherCAT PDO Transmit   Priority=3  sig_name=Box 8 (YISUWORLD).Setpoint Values process data mapping.ResValue3  sig_offset=12528  sig_type=uint16  type_size=16  sig_dim=1  device_id=0  sample_time=0.001000
      settings: SourceProductBaseCode=XP
  EtherCAT PDO Transmit RES CH4 : xpcethercatlib/EtherCAT PDO Transmit   Priority=3  sig_name=Box 8 (YISUWORLD).Setpoint Values process data mapping.ResValue4  sig_offset=12544  sig_type=uint16  type_size=16  sig_dim=1  device_id=0  sample_time=0.001000
      settings: SourceProductBaseCode=XP
  EtherCAT PDO Transmit RES CH5 : xpcethercatlib/EtherCAT PDO Transmit   Priority=3  sig_name=Box 8 (YISUWORLD).Setpoint Values process data mapping.ResValue5  sig_offset=12560  sig_type=uint16  type_size=16  sig_dim=1  device_id=0  sample_time=0.001000
      settings: SourceProductBaseCode=XP
  EtherCAT PDO Transmit RES CH6 : xpcethercatlib/EtherCAT PDO Transmit   Priority=3  sig_name=Box 8 (YISUWORLD).Setpoint Values process data mapping.ResValue6  sig_offset=12576  sig_type=uint16  type_size=16  sig_dim=1  device_id=0  sample_time=0.001000
      settings: SourceProductBaseCode=XP
  EtherCAT PDO Transmit RES CH7 : xpcethercatlib/EtherCAT PDO Transmit   Priority=3  sig_name=Box 8 (YISUWORLD).Setpoint Values process data mapping.ResValue7  sig_offset=12592  sig_type=uint16  type_size=16  sig_dim=1  device_id=0  sample_time=0.001000
      settings: SourceProductBaseCode=XP
  EtherCAT PDO Transmit RES CH8 : xpcethercatlib/EtherCAT PDO Transmit   Priority=3  sig_name=Box 8 (YISUWORLD).Setpoint Values process data mapping.ResValue8  sig_offset=12608  sig_type=uint16  type_size=16  sig_dim=1  device_id=0  sample_time=0.001000
      settings: SourceProductBaseCode=XP
  EtherCAT PDO Transmit RES CH9 : xpcethercatlib/EtherCAT PDO Transmit   Priority=3  sig_name=Box 8 (YISUWORLD).Setpoint Values process data mapping.ResValue9  sig_offset=12624  sig_type=uint16  type_size=16  sig_dim=1  device_id=0  sample_time=0.001000
      settings: SourceProductBaseCode=XP
  wires:
  Res_CH1/1 -> DTCB CH1/1
  DTCB CH1/1 -> EtherCAT PDO Transmit RES CH1/1
  Res_CH2/1 -> DTCB CH2/1
  DTCB CH2/1 -> EtherCAT PDO Transmit RES CH2/1
  Res_CH3/1 -> DTCB CH3/1
  DTCB CH3/1 -> EtherCAT PDO Transmit RES CH3/1
  Res_CH4/1 -> DTCB CH4/1
  DTCB CH4/1 -> EtherCAT PDO Transmit RES CH4/1
  Res_CH5/1 -> DTCB CH5/1
  DTCB CH5/1 -> EtherCAT PDO Transmit RES CH5/1
  Res_CH6/1 -> DTCB CH6/1
  DTCB CH6/1 -> EtherCAT PDO Transmit RES CH6/1
  Res_CH7/1 -> DTCB CH7/1
  DTCB CH7/1 -> EtherCAT PDO Transmit RES CH7/1
  Res_CH8/1 -> DTCB CH8/1
  DTCB CH8/1 -> EtherCAT PDO Transmit RES CH8/1
  Res_CH9/1 -> DTCB CH9/1
  DTCB CH9/1 -> EtherCAT PDO Transmit RES CH9/1
  Res_CH10/1 -> DTCB CH10/1
  DTCB CH10/1 -> EtherCAT PDO Transmit RES CH10/1
  Res_CH11/1 -> DTCB CH11/1
  DTCB CH11/1 -> EtherCAT PDO Transmit RES CH11/1
  Res_CH12/1 -> DTCB CH12/1
  DTCB CH12/1 -> EtherCAT PDO Transmit RES CH12/1

== system EHB_speedgoat_R2020a_V1/保留/TIF_02/CB3012_01/Res2Cmd ==
  ResVal : Inport
  Add : Sum  Inputs=-+
  Constant : Constant
  Divide : Product  Inputs=*/  OutDataTypeStr=uint16  RndMeth=Round
  MaxResVal : Constant  Value=1e6  OutDataTypeStr=Inherit: Inherit via back propagation
  Switch : Switch  Criteria=u2 > Threshold  OutDataTypeStr=Inherit: Inherit via back propagation
  zero : Constant  Value=0  OutDataTypeStr=Inherit: Inherit via back propagation
  CmdVal : Outport
  wires:
  MaxResVal/1 -> Divide/1
  Divide/1 -> Switch/1
  Switch/1 -> CmdVal/1
  zero/1 -> Switch/3
  ResVal/1 -> Add/2
  Add/1 -> Divide/2, Switch/2
  Constant/1 -> Add/1

== system EHB_speedgoat_R2020a_V1/保留/TIF_02/CB3012_01/Res2Cmd1 ==
  ResVal : Inport
  Add : Sum  Inputs=-+
  Constant : Constant
  Divide : Product  Inputs=*/  OutDataTypeStr=uint16  RndMeth=Round
  MaxResVal : Constant  Value=1e6  OutDataTypeStr=Inherit: Inherit via back propagation
  Switch : Switch  Criteria=u2 > Threshold  OutDataTypeStr=Inherit: Inherit via back propagation
  zero : Constant  Value=0  OutDataTypeStr=Inherit: Inherit via back propagation
  CmdVal : Outport
  wires:
  Constant/1 -> Add/1
  Add/1 -> Switch/2, Divide/2
  ResVal/1 -> Add/2
  zero/1 -> Switch/3
  Switch/1 -> CmdVal/1
  Divide/1 -> Switch/1
  MaxResVal/1 -> Divide/1

== system EHB_speedgoat_R2020a_V1/保留/TIF_02/CB3012_01/Res2Cmd10 ==
  ResVal : Inport
  Add : Sum  Inputs=-+
  Constant : Constant
  Divide : Product  Inputs=*/  OutDataTypeStr=uint16  RndMeth=Round
  MaxResVal : Constant  Value=1e6  OutDataTypeStr=Inherit: Inherit via back propagation
  Switch : Switch  Criteria=u2 > Threshold  OutDataTypeStr=Inherit: Inherit via back propagation
  zero : Constant  Value=0  OutDataTypeStr=Inherit: Inherit via back propagation
  CmdVal : Outport
  wires:
  MaxResVal/1 -> Divide/1
  Divide/1 -> Switch/1
  Switch/1 -> CmdVal/1
  zero/1 -> Switch/3
  ResVal/1 -> Add/2
  Add/1 -> Divide/2, Switch/2
  Constant/1 -> Add/1

== system EHB_speedgoat_R2020a_V1/保留/TIF_02/CB3012_01/Res2Cmd11 ==
  ResVal : Inport
  Add : Sum  Inputs=-+
  Constant : Constant
  Divide : Product  Inputs=*/  OutDataTypeStr=uint16  RndMeth=Round
  MaxResVal : Constant  Value=1e6  OutDataTypeStr=Inherit: Inherit via back propagation
  Switch : Switch  Criteria=u2 > Threshold  OutDataTypeStr=Inherit: Inherit via back propagation
  zero : Constant  Value=0  OutDataTypeStr=Inherit: Inherit via back propagation
  CmdVal : Outport
  wires:
  Constant/1 -> Add/1
  Add/1 -> Switch/2, Divide/2
  ResVal/1 -> Add/2
  zero/1 -> Switch/3
  Switch/1 -> CmdVal/1
  Divide/1 -> Switch/1
  MaxResVal/1 -> Divide/1

== system EHB_speedgoat_R2020a_V1/保留/TIF_02/CB3012_01/Res2Cmd2 ==
  ResVal : Inport
  Add : Sum  Inputs=-+
  Constant : Constant
  Divide : Product  Inputs=*/  OutDataTypeStr=uint16  RndMeth=Round
  MaxResVal : Constant  Value=1e6  OutDataTypeStr=Inherit: Inherit via back propagation
  Switch : Switch  Criteria=u2 > Threshold  OutDataTypeStr=Inherit: Inherit via back propagation
  zero : Constant  Value=0  OutDataTypeStr=Inherit: Inherit via back propagation
  CmdVal : Outport
  wires:
  MaxResVal/1 -> Divide/1
  Divide/1 -> Switch/1
  Switch/1 -> CmdVal/1
  zero/1 -> Switch/3
  ResVal/1 -> Add/2
  Add/1 -> Divide/2, Switch/2
  Constant/1 -> Add/1

== system EHB_speedgoat_R2020a_V1/保留/TIF_02/CB3012_01/Res2Cmd3 ==
  ResVal : Inport
  Add : Sum  Inputs=-+
  Constant : Constant
  Divide : Product  Inputs=*/  OutDataTypeStr=uint16  RndMeth=Round
  MaxResVal : Constant  Value=1e6  OutDataTypeStr=Inherit: Inherit via back propagation
  Switch : Switch  Criteria=u2 > Threshold  OutDataTypeStr=Inherit: Inherit via back propagation
  zero : Constant  Value=0  OutDataTypeStr=Inherit: Inherit via back propagation
  CmdVal : Outport
  wires:
  Constant/1 -> Add/1
  Add/1 -> Switch/2, Divide/2
  ResVal/1 -> Add/2
  zero/1 -> Switch/3
  Switch/1 -> CmdVal/1
  Divide/1 -> Switch/1
  MaxResVal/1 -> Divide/1

== system EHB_speedgoat_R2020a_V1/保留/TIF_02/CB3012_01/Res2Cmd4 ==
  ResVal : Inport
  Add : Sum  Inputs=-+
  Constant : Constant
  Divide : Product  Inputs=*/  OutDataTypeStr=uint16  RndMeth=Round
  MaxResVal : Constant  Value=1e6  OutDataTypeStr=Inherit: Inherit via back propagation
  Switch : Switch  Criteria=u2 > Threshold  OutDataTypeStr=Inherit: Inherit via back propagation
  zero : Constant  Value=0  OutDataTypeStr=Inherit: Inherit via back propagation
  CmdVal : Outport
  wires:
  MaxResVal/1 -> Divide/1
  Divide/1 -> Switch/1
  Switch/1 -> CmdVal/1
  zero/1 -> Switch/3
  ResVal/1 -> Add/2
  Add/1 -> Divide/2, Switch/2
  Constant/1 -> Add/1

== system EHB_speedgoat_R2020a_V1/保留/TIF_02/CB3012_01/Res2Cmd5 ==
  ResVal : Inport
  Add : Sum  Inputs=-+
  Constant : Constant
  Divide : Product  Inputs=*/  OutDataTypeStr=uint16  RndMeth=Round
  MaxResVal : Constant  Value=1e6  OutDataTypeStr=Inherit: Inherit via back propagation
  Switch : Switch  Criteria=u2 > Threshold  OutDataTypeStr=Inherit: Inherit via back propagation
  zero : Constant  Value=0  OutDataTypeStr=Inherit: Inherit via back propagation
  CmdVal : Outport
  wires:
  Constant/1 -> Add/1
  Add/1 -> Switch/2, Divide/2
  ResVal/1 -> Add/2
  zero/1 -> Switch/3
  Switch/1 -> CmdVal/1
  Divide/1 -> Switch/1
  MaxResVal/1 -> Divide/1
